simulink model "Copy_of_controllo_ss_PP_Luenberger"  (R2023b)
settings: Solver=VariableStepAuto  StartTime=0.0  StopTime=10  RelTol=1e-3
values from neighbouring files (symbols this model uses):
  A_ob = A - L_kf*C    [LQ_KF_version1.m]    (also in LQ_KF_version2.m; LQ_Luenberger.m; PP_Luenberger.m = A - L*C; prova1.m = A - L*C)
  B_ob = [ B - L_kf*D, L_kf]    [LQ_KF_version1.m]    (also in LQ_KF_version2.m; LQ_Luenberger.m; PP_Luenberger.m = [ B, L]; prova1.m = [ B, L])
  C_ob = eye(n)    [LQ_KF_version1.m]    (also in LQ_KF_version2.m; LQ_Luenberger.m; PP_Luenberger.m; prova1.m)
  D_ob = zeros(n, m+p)    [LQ_KF_version1.m]    (also in LQ_KF_version2.m; LQ_Luenberger.m; PP_Luenberger.m; prova1.m)
  Ken_eta = K(:, 4)    [LQ_KF_version1.m]    (also in LQ_KF_version2.m = Ken(:, n+1:end); LQ_Luenberger.m; PP_Luenberger.m = Ken(:, n+1:end); prova1.m = Ken(:, n+1:end))
  Ken_x = K(:, 1:3)    [LQ_KF_version1.m]    (also in LQ_KF_version2.m = Ken(:, 1:n); LQ_Luenberger.m; PP_Luenberger.m = Ken(:, 1:n); prova1.m = Ken(:, 1:n))
  m = 1    [LQ_KF_version1.m]    (also in LQ_KF_version2.m; LQ_Luenberger.m; PP_Luenberger.m; prova1.m)
undefined symbols (not defined in the file or in its folder): A, B, C, D, k_mag, Lc, Rtot, x1_eq0, x2_eq0, y0
settings Model: Creator=Pronto all'uso  LastModifiedBy=lollo

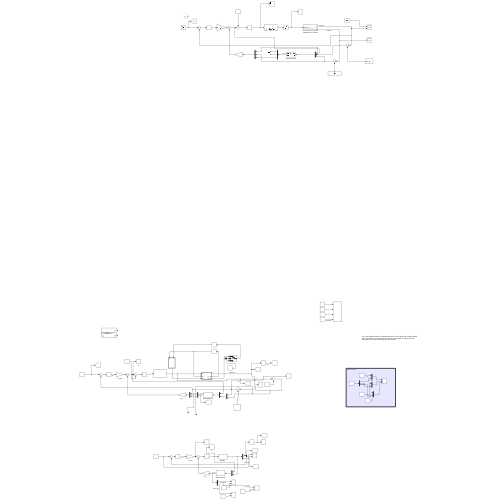
[thumbnail: Simulink's stored preview of the top-level diagram]
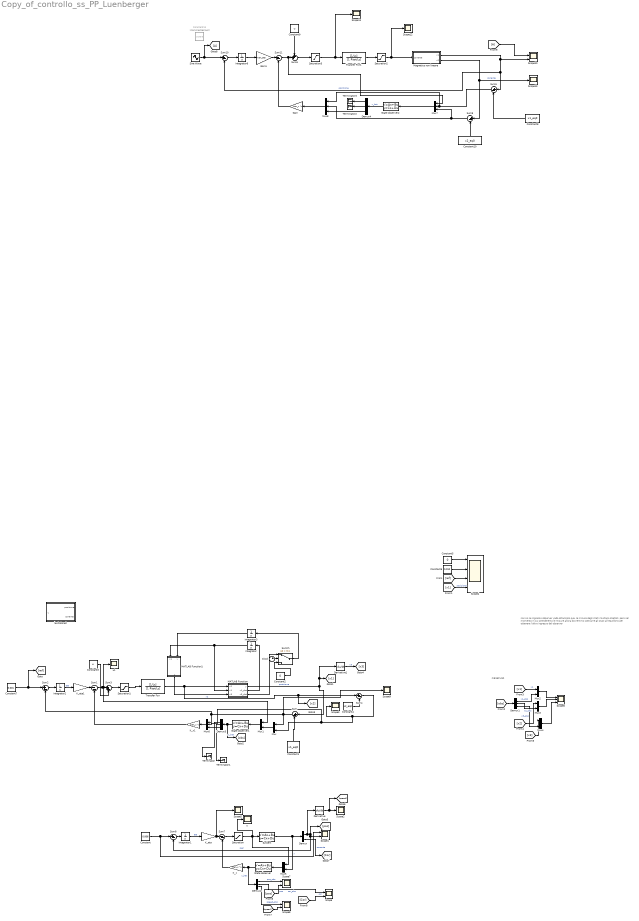
== system Copy_of_controllo_ss_PP_Luenberger ==
  note: OBSERVER
  note: non so se ingresso observer vada attaccato qua. le misure degli stati risultano sballati. pero nel momento in cui prenderemo le misure allora dovremmo sottrarre gli stati all'equilibrio per ottenere l'altro ingresso del observer
  Clock : Clock
  Constant : Constant  Value=0.006
  Constant1 : Constant  Value=x1_eq0
  Constant10 : Constant  Value=x2_eq0
  Constant11 : Constant  Commented=on  Value=3.5e-3
  Constant2 : Constant  Value=0
  Constant3 : Constant  Value=u
  Constant4 : Constant  Value=x2_eq0
  Constant5 : Constant  Value=0
  Constant6 : Constant  Value=0.012
  Constant7 : Constant  Value=0.001
  Constant8 : Constant  Value=x1_eq0
  Constant9 : Constant  Value=u
  Demux : Demux  Outputs=2
  Demux{1..4} (4 alike) : Demux  Outputs=3
  Derivative : Derivative
  Derivative1 : Derivative
  From9 : From
  Gain : Gain  Gain=Ken_x  Multiplication=Matrix(K*u)
  Gain1 : Gain  Gain=Ken_eta
  Goto8 : Goto
  Integrator{,1..3,6} (5 alike) : Integrator
  K_eta : Gain  Gain=Ken_eta  Multiplication=Matrix(K*u) (u vector)
  K_eta1 : Gain  Gain=Ken_eta  Multiplication=Matrix(K*u) (u vector)
  K_x : Gain  Gain=Ken_x  Multiplication=Matrix(K*u) (u vector)
  K_x1 : Gain  Gain=Ken_x  Multiplication=Matrix(K*u) (u vector)
  MATLAB Function : MATLAB Function  TreatAsAtomicUnit=on
  MATLAB Function1 : MATLAB Function  TreatAsAtomicUnit=on
  Magnetico non lineare : Subsystem
  Mux{,1..5} (6 alike) : Mux  Inputs=2
  Mux6 : Mux  Inputs=3
  Mux7 : Mux  Inputs=3
  Mux8 : Mux  Inputs=3
  Saturation : Saturate  UpperLimit=23  LowerLimit=-23
  Saturation1 : Saturate  UpperLimit=23  LowerLimit=0
  Saturation2 : Saturate  UpperLimit=3  LowerLimit=0
  Saturation3 : Saturate  UpperLimit=24  LowerLimit=-24
  Scope{,1,7..8,10} (5 alike) : Scope  NumInputPorts=2
  Scope{2..3,5,9,11..13} (7 alike) : Scope
  Scope4 : Scope  NumInputPorts=4
  Scope6 : Scope  NumInputPorts=3
  Sine Wave : Sin  Amplitude=0.002  Bias=0.004  Frequency=10  SampleTime=0
  State observer : StateSpace  A=A_ob  B=B_ob  C=C_ob  D=D_ob  InitialCondition=[0.002;0;0]  ParameterTunability=Unconstrained
  State observer1 : StateSpace  A=A_ob  B=B_ob  C=C_ob  D=D_ob  InitialCondition=[0;0;0]  ParameterTunability=Unconstrained
  State observer2 : StateSpace  A=A_ob  B=B_ob  C=C_ob  D=D_ob  InitialCondition=[0;0;0]  ParameterTunability=Unconstrained
  Sum{,2,4..5,8..10} (7 alike) : Sum  Inputs=|+-
  Sum1 : Sum  Inputs=|--
  Sum11 : Sum  Inputs=|--
  Sum3 : Sum  Inputs=|++
  Sum6 : Sum  Inputs=++|
  Sum7 : Sum  Inputs=|--
  Switch : Switch  Criteria=u2 > Threshold  Threshold=0.1  SaturateOnIntegerOverflow=off  InputSameDT=off
  System : StateSpace  A=A  B=B  C=C  D=D  InitialCondition=[0; 0;0]  ParameterTunability=Unconstrained
  Terminator{,1..3} (4 alike) : Terminator
  Transfer Fcn : TransferFcn  Numerator=[1/Lc]  Denominator=[1 Rtot/Lc]
  Transfer Fcn1 : TransferFcn  Numerator=[1/Lc]  Denominator=[1 Rtot/Lc]
  levitatore2 : Subsystem  Description=|  mask{y1_0=0, y2_0=0}
      | Magnetic Levitation System.
      | The input is the squared current. The outputs are the position (y1) and the velocity (y2).
      mask prompts: y1_0 "Initial value for y1"; y2_0 "Initial value for y2"
      mask DialogControl DescTextVar Prompt: Magnetic Levitation System. The input is the squared current. The outputs are the position (y1) and the velocity (y2).
      mask Display:
      | disp('Magnetic Levitation\nSystem');
      | port_label('input', 1, 'i= i\_tilde^2', 'texmode', 'on');
      | port_label('output', 1, 'y_1');
      | port_label('output', 2, 'y_2');
  u : Scope
  u1 : Scope
  wires:
  Integrator1/1 -> K_eta/1  "eta"
  K_x/1 -> Sum7/2
  Sum8/1 -> Integrator1/1
  K_eta/1 -> Scope5/1, Sum7/1
  System/1 -> Demux/1, Mux5/2  "y"
  State observer/1 -> Demux2/1, K_x/1  "x_hat"
  Mux5/1 -> State observer/1
  Demux/1 -> Derivative/1, [pos], Scope1/2, Sum8/2  "real"
  Demux/2 -> [Cor]  "corrente"
  Constant/1 -> Scope1/1, Sum8/1
  Sum7/1 -> Saturation/1
  Saturation/1 -> Mux5/1, u/1, System/1
  Derivative/1 -> [speed], Scope2/1
  State observer1/1 -> Demux3/1, [obs]  "x_hat"
  Sum2/1 -> Integrator2/1
  Integrator2/1 -> K_eta1/1  "eta"
  Sum1/1 -> u1/1, Mux1/1, Sum3/1
  K_eta1/1 -> Sum1/1
  K_x1/1 -> Sum1/2
  Constant7/1 -> [ref], Sum2/1
  Mux1/1 -> State observer1/1
  [ref] -> Scope4/3
  Constant5/1 -> Scope4/1
  Constant6/1 -> Scope4/2
  Transfer Fcn/1 -> Sum4/1, [x2], MATLAB Function/1(x2)  "x2"
  MATLAB Function/1(y) -> Sum/1, [x1], Derivative1/1  "posizione"
  [x1] -> Scope4/4  "posizione"
  [obs] -> Demux1/1
  [x1] -> Mux2/1  "x1"
  Demux1/1 -> Mux2/2  "x1_obs"
  Demux1/2 -> Mux3/2  "x2_obs"
  [x2] -> Mux3/1
  Mux3/1 -> Scope6/2
  Mux2/1 -> Scope6/1
  Demux1/3 -> Mux4/2  "x3_obs"
  Derivative1/1 -> [x3]  "x3"
  [x3] -> Mux4/1
  Mux4/1 -> Scope6/3
  Demux2/1 -> Scope7/1  "pos_obs"
  [pos] -> Scope7/2  "pos"
  Demux2/3 -> Scope8/1  "speed_obs"
  [speed] -> Scope8/2
  Demux2/2 -> Scope/1  "cor_obs"
  [Cor] -> Scope/2  "cor"
  Sum/1 -> Scope9/1, Mux/1, Mux6/1, Sum2/2
  Constant1/1 -> Sum/2
  Constant3/1 -> Sum3/2
  Sum3/1 -> Saturation1/1
  Constant4/1 -> Sum4/2
  Mux/1 -> Mux1/2
  Sum4/1 -> Mux6/2, Mux/2, Scope3/1
  Saturation1/1 -> Transfer Fcn/1
  Demux3/1 -> Terminator/1
  Demux3/2 -> Terminator1/1
  Mux6/1 -> K_x1/1
  Demux3/3 -> Mux6/3
  MATLAB Function/3(x3_dot) -> Switch/1
  MATLAB Function1/1(y) -> MATLAB Function/3(x3)
  Integrator3/1 -> MATLAB Function1/2(v)
  MATLAB Function/2(x1_dot) -> Integrator/1
  Integrator/1 -> MATLAB Function/2(x1), MATLAB Function1/1(x1)
  Constant2/1 -> Switch/3
  Clock/1 -> Switch/2
  Switch/1 -> Integrator3/1
  Transfer Fcn1/1 -> Saturation2/1
  Saturation2/1 -> Magnetico non lineare/1(corrente), Scope12/1
  Magnetico non lineare/1(x1) -> Sum10/2, Sum5/1, Scope10/2  "posizione"
  Constant8/1 -> Sum5/2
  Sum6/1 -> Saturation3/1
  Constant9/1 -> Sum6/1
  Mux7/1 -> State observer2/1
  Sum5/1 -> Mux8/1, Mux7/2
  Constant10/1 -> Sum9/2
  Sum9/1 -> Mux8/2, Mux7/3
  Gain1/1 -> Sum11/1
  Gain/1 -> Sum11/2
  Integrator6/1 -> Gain1/1
  Sum10/1 -> Integrator6/1
  Magnetico non lineare/2(x2) -> Sum9/1, Scope13/1  "corrente"
  Sum11/1 -> Mux7/1, Sum6/2
  Saturation3/1 -> Transfer Fcn1/1, Scope11/1
  State observer2/1 -> Demux4/1  "x_hat"
  Mux8/1 -> Gain/1
  Demux4/3 -> Mux8/3
  Demux4/1 -> Terminator3/1
  Demux4/2 -> Terminator2/1
  Sine Wave/1 -> Goto8/1, Sum10/1
  From9/1 -> Scope10/1

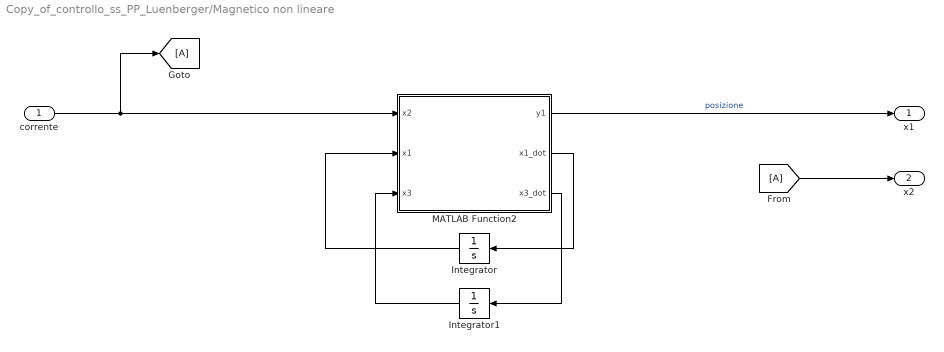
== system Copy_of_controllo_ss_PP_Luenberger/Magnetico non lineare ==
  corrente : Inport
  From : From
  Goto : Goto
  Integrator : Integrator
  Integrator1 : Integrator
  MATLAB Function2 : MATLAB Function  TreatAsAtomicUnit=on
  x1 : Outport
  x2 : Outport  Port=2
  wires:
  corrente/1 -> Goto/1, MATLAB Function2/1(x2)
  MATLAB Function2/1(y1) -> x1/1  "posizione"
  MATLAB Function2/2(x1_dot) -> Integrator/1
  Integrator/1 -> MATLAB Function2/2(x1)
  MATLAB Function2/3(x3_dot) -> Integrator1/1
  Integrator1/1 -> MATLAB Function2/3(x3)
  From/1 -> x2/1

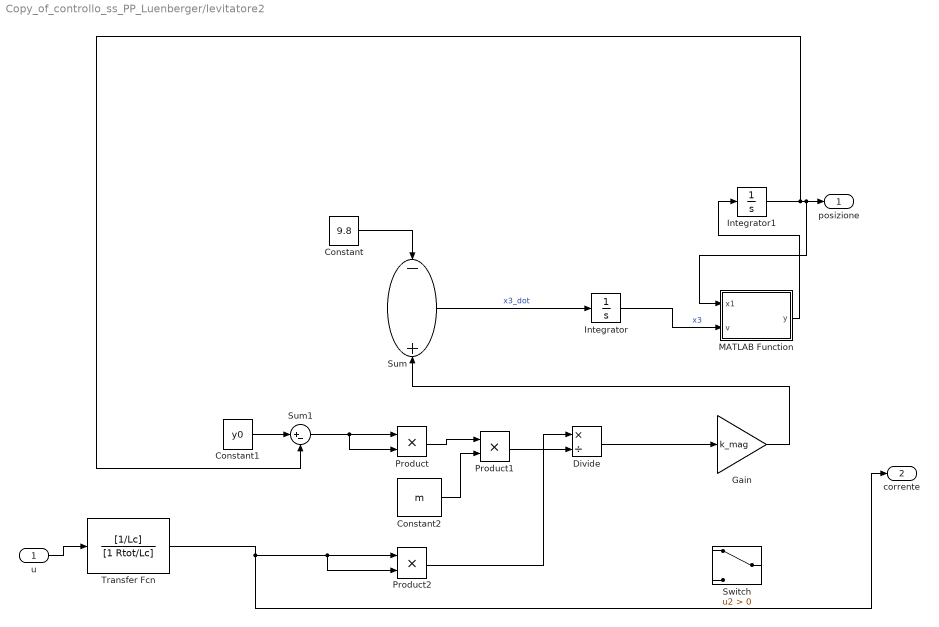
== system Copy_of_controllo_ss_PP_Luenberger/levitatore2 ==
  u : Inport
  Constant : Constant  Value=9.8
  Constant1 : Constant  Value=y0
  Constant2 : Constant  Value=m
  Divide : Product  Inputs=*/
  Gain : Gain  Gain=k_mag
  Integrator : Integrator  InitialCondition=y2_0
  Integrator1 : Integrator  InitialCondition=y1_0
  MATLAB Function : MATLAB Function  TreatAsAtomicUnit=on
  Product : Product  RndMeth=Zero
  Product1 : Product  RndMeth=Zero
  Product2 : Product
  Sum : Sum  Inputs=-+
  Sum1 : Sum  Inputs=|+-
  Switch : Switch  Criteria=u2 > Threshold  SaturateOnIntegerOverflow=off  InputSameDT=off
  Transfer Fcn : TransferFcn  Numerator=[1/Lc]  Denominator=[1 Rtot/Lc]
  posizione : Outport
  corrente : Outport  Port=2
  wires:
  Integrator/1 -> MATLAB Function/2(v)  "x3"
  Constant1/1 -> Sum1/1
  Integrator1/1 -> MATLAB Function/1(x1), posizione/1, Sum1/2
  Sum/1 -> Integrator/1  "x3_dot"
  Constant2/1 -> Product1/2
  Sum1/1 -> Product/1, Product/2
  Product/1 -> Product1/1
  Constant/1 -> Sum/1
  u/1 -> Transfer Fcn/1
  Transfer Fcn/1 -> corrente/1, Product2/2, Product2/1
  Product2/1 -> Divide/1
  Product1/1 -> Divide/2
  Divide/1 -> Gain/1
  Gain/1 -> Sum/2
  MATLAB Function/1(y) -> Integrator1/1

== matlab function Copy_of_controllo_ss_PP_Luenberger/levitatore2/MATLAB Function ==
  data: x1 input; y output; v input
function y = fcn(x1, v)
    if x1 <= 0 && v > 0
        v = 0
    end

y = v;

== matlab function Copy_of_controllo_ss_PP_Luenberger/MATLAB Function ==
  data: y output; x2 input; x1_dot output; x1 input; x3 input; x3_dot output
function [y,x1_dot, x3_dot] = fcn(x2, x1, x3)
    m = 0.0657;
    g = 9.81;
    k_mag = 2.4405e-05;
    Rtot = 9.7585;
    Lc = 0.3708;
    y0 = 0.012;
    
    x1_dot = x3;
    x3_dot = (k_mag/m)*(x2/(y0-x1))^2 - g;
y = x1;

== matlab function Copy_of_controllo_ss_PP_Luenberger/MATLAB Function1 ==
  data: x1 input; y output; v input
function y = fcn(x1, v)
    if x1 <= 0 && v > 0
        v = 0
    end

y = v;

== matlab function Copy_of_controllo_ss_PP_Luenberger/Magnetico non lineare/MATLAB Function2 ==
  data: y1 output; x2 input; x1_dot output; x1 input; x3 input; x3_dot output
function [y1,x1_dot, x3_dot] = fcn(x2, x1, x3)
    m = 0.0657;
    g = 9.81;
    k_mag = 2.4405e-05;
    Rtot = 9.7585;
    Lc = 0.3708;
    y0 = 0.012;
    
    x1_dot = x3;
    if x1 < y0
        x3_dot = (k_mag/m)*(x2/(y0-x1))^2 - g;
    else
        x1 = 0.012;
        x3_dot = 0;
        x3 = 0;
    end

    
    % condizioni
    if x1 <=0 && x3_dot < 0
        x1 = 0;
        x3 = 0;
        x3_dot = 0;
    end
y1 = x1;
